simulink model "fivebitadder_final"  (R2020b)
settings: Solver=VariableStepAuto  StartTime=0.0  StopTime=1  RelTol=1e-3
libraries: commutil2 x3
settings Model: Creator=ansha  LastModifiedBy=Aniket Singh
settings SFSimCC: CustomCodeUndefinedFunction=UseInterfaceOnly

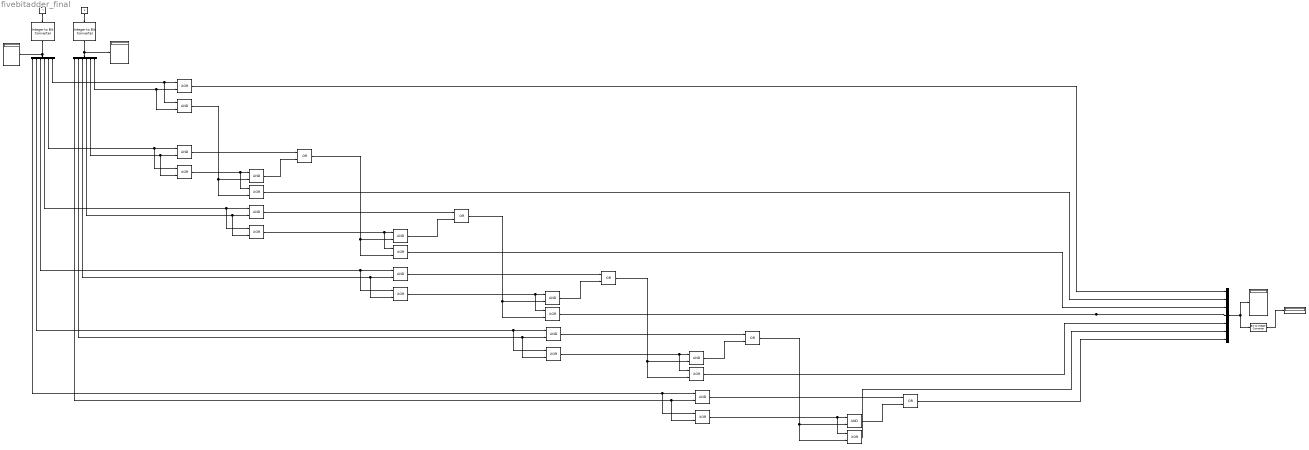
== system fivebitadder_final ==
  Bit to Integer Converter : commutil2/Bit to Integer Converter  nbits=7  bitOrder=LSB first  signedOutputValues=Unsigned  outDtype=Inherit via internal rule  outDtypeSigned=Inherit via internal rule
  Bus Creator : BusCreator  DialogController=Simulink.DDGSource_BusCreator  Inputs=7
  Constant12 : Constant  Value=7
  Constant13 : Constant  Value=5
  Demux1 : Demux  Outputs=6
  Demux2 : Demux  Outputs=6
  Display{,7..9} (4 alike) : Display
  Integer to Bit Converter : commutil2/Integer to Bit Converter  nbits=6  signedInputValues=Unsigned  bitOrder=MSB first  outDtype=Inherit via internal rule
  Integer to Bit Converter1 : commutil2/Integer to Bit Converter  nbits=6  signedInputValues=Unsigned  bitOrder=MSB first  outDtype=Inherit via internal rule
  Logical Operator{,2,5,7,9,12,16..17,21..22,26} (11 alike) : Logic  AllPortsSameDT=off  OutDataTypeStr=boolean
  Logical Operator{1,3,6,8,10,13..14,18..19,23..24} (11 alike) : Logic  Operator=XOR  AllPortsSameDT=off  OutDataTypeStr=boolean
  Logical Operator{4,11,15,20,25} (5 alike) : Logic  Operator=OR  AllPortsSameDT=off  OutDataTypeStr=boolean
  wires:
  Demux1/5 -> Logical Operator1/1, Logical Operator/1
  Demux2/5 -> Logical Operator/2, Logical Operator1/2
  Logical Operator1/1 -> Logical Operator3/1, Logical Operator2/1
  Logical Operator/1 -> Logical Operator4/1
  Logical Operator2/1 -> Logical Operator4/2
  Logical Operator3/1 -> Bus Creator/2
  Demux1/6 -> Logical Operator6/1, Logical Operator5/1
  Demux2/6 -> Logical Operator5/2, Logical Operator6/2
  Logical Operator5/1 -> Logical Operator3/2, Logical Operator2/2
  Logical Operator6/1 -> Bus Creator/1
  Demux1/4 -> Logical Operator8/1, Logical Operator7/1
  Demux2/4 -> Logical Operator7/2, Logical Operator8/2
  Logical Operator7/1 -> Logical Operator11/1
  Logical Operator8/1 -> Logical Operator10/1, Logical Operator9/1
  Logical Operator10/1 -> Bus Creator/3
  Logical Operator9/1 -> Logical Operator11/2
  Logical Operator4/1 -> Logical Operator9/2, Logical Operator10/2
  Demux1/3 -> Logical Operator13/1, Logical Operator12/1
  Demux2/3 -> Logical Operator12/2, Logical Operator13/2
  Logical Operator16/1 -> Logical Operator15/2
  Logical Operator14/1 -> Bus Creator/4
  Logical Operator12/1 -> Logical Operator15/1
  Logical Operator13/1 -> Logical Operator14/1, Logical Operator16/1
  Logical Operator11/1 -> Logical Operator14/2, Logical Operator16/2
  Logical Operator18/1 -> Logical Operator19/1, Logical Operator21/1
  Logical Operator17/1 -> Logical Operator20/1
  Logical Operator21/1 -> Logical Operator20/2
  Demux1/2 -> Logical Operator18/1, Logical Operator17/1
  Demux2/2 -> Logical Operator17/2, Logical Operator18/2
  Logical Operator15/1 -> Logical Operator19/2, Logical Operator21/2
  Demux1/1 -> Logical Operator23/1, Logical Operator22/1
  Demux2/1 -> Logical Operator22/2, Logical Operator23/2
  Logical Operator24/1 -> Bus Creator/6
  Logical Operator26/1 -> Logical Operator25/2
  Logical Operator22/1 -> Logical Operator25/1
  Logical Operator23/1 -> Logical Operator24/1, Logical Operator26/1
  Logical Operator20/1 -> Logical Operator24/2, Logical Operator26/2
  Logical Operator25/1 -> Bus Creator/7
  Constant12/1 -> Integer to Bit Converter/1
  Integer to Bit Converter/1 -> Demux1/1, Display9/1
  Constant13/1 -> Integer to Bit Converter1/1
  Integer to Bit Converter1/1 -> Display8/1, Demux2/1
  Logical Operator19/1 -> Bus Creator/5
  Bus Creator/1 -> Display/1, Bit to Integer Converter/1
  Bit to Integer Converter/1 -> Display7/1
